simulink model "model_3_transfer_fcn"  (R2021b)
settings: Solver=FixedStepAuto  StartTime=0.0  StopTime=1  FixedStep=0.00005  RelTol=1e-3
settings Model: Creator=den  LastModifiedBy=den

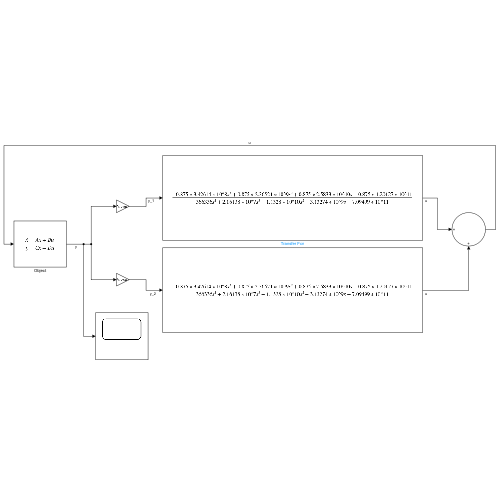
[thumbnail: Simulink's stored preview of the top-level diagram]
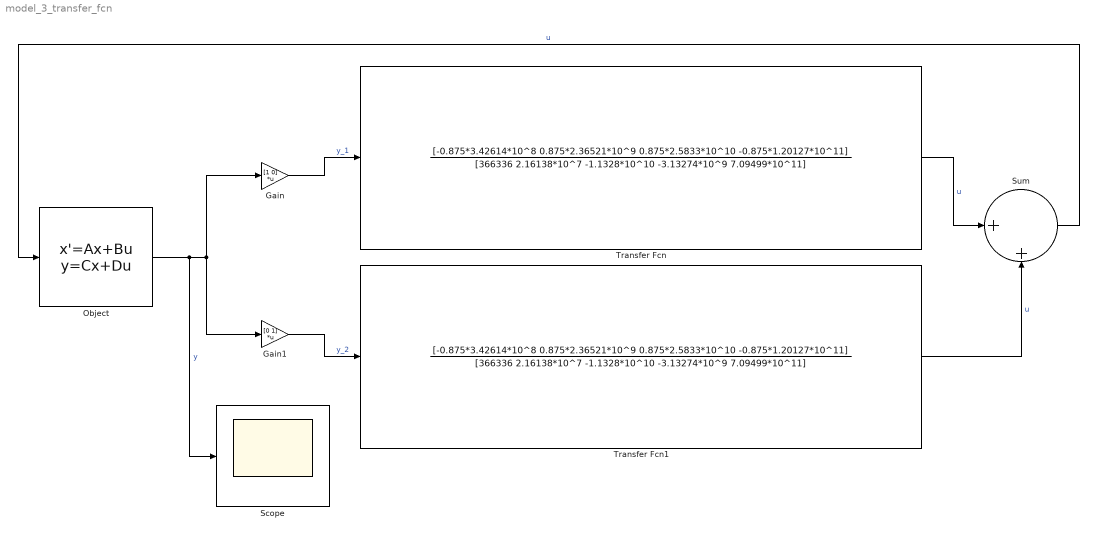
== system model_3_transfer_fcn ==
  Gain : Gain  Gain=[1 0]  Multiplication=Matrix(K*u) (u vector)
  Gain1 : Gain  Gain=[0 1]  Multiplication=Matrix(K*u) (u vector)
  Object : StateSpace  A=[5 -7 -5 1; -7 5 -1 5; -5 -1 5 7; 1 5 7 5]  B=[5; 7; 1; 9]  C=[0 0 2 2; 1 1 -1 1]  D=[0;0]  InitialCondition=[28; -14; 2; -19]
  Scope : Scope
  Sum : Sum  Inputs=|++
  Transfer Fcn : TransferFcn  Numerator=[-0.875*3.42614*10^8 0.875*2.36521*10^9 0.875*2.5833*10^10 -0.875*1.20127*10^11]  Denominator=[366336 2.16138*10^7 -1.1328*10^10 -3.13274*10^9 7.09499*10^11]
  Transfer Fcn1 : TransferFcn  Numerator=[-0.875*3.42614*10^8 0.875*2.36521*10^9 0.875*2.5833*10^10 -0.875*1.20127*10^11]  Denominator=[366336 2.16138*10^7 -1.1328*10^10 -3.13274*10^9 7.09499*10^11]
  wires:
  Object/1 -> Scope/1, Gain/1, Gain1/1  "y"
  Gain/1 -> Transfer Fcn/1  "y_1"
  Gain1/1 -> Transfer Fcn1/1  "y_2"
  Transfer Fcn1/1 -> Sum/2  "u"
  Transfer Fcn/1 -> Sum/1  "u"
  Sum/1 -> Object/1  "u"
